simulink subsystem "DCDCConverter"  (R2024b)
settings: Solver=VariableStepAuto  StartTime=0.0  StopTime=10.0  RelTol=1e-3
undefined symbols (not defined in the file): PlntDCDCMass, PlntDCDCVoltInit, PlntEMCp
libraries: autolibutils x1, autolibdcdc x1, autolibsharedcommon x1
settings Model: ModifiedByFormat=The MathWorks, Inc.  Creator=The MathWorks, Inc.  LastModifiedBy=The MathWorks, Inc.
settings OptimizationCC: ReuseModelBlockBuffer=off
settings RTWCC: GPUComputeCapability=3.5

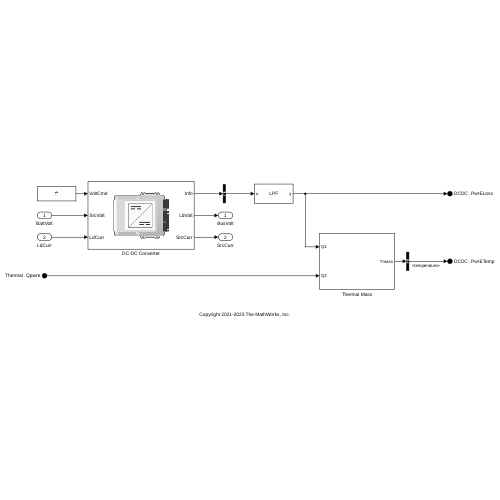
[thumbnail: Simulink's stored preview of the top-level diagram]
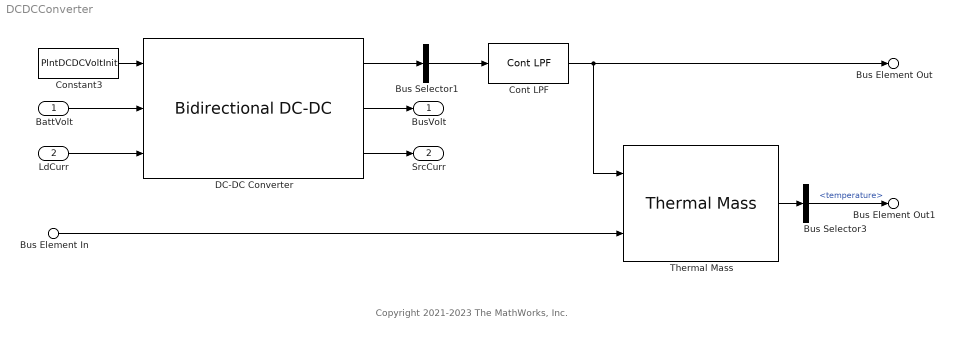
== system DCDCConverter ==
  note: Copyright 2021-2023 The MathWorks, Inc.
  BattVolt : Inport
  LdCurr : Inport  Port=2
  Bus Element In : Inport  Port=3  PortName=Thermal  Element=Qpwre
  Bus Selector1 : BusSelector  OutputSignals=PwrLoss  OutputAsBus=on
  Bus Selector3 : BusSelector  OutputSignals=temperature
  Constant3 : Constant  Value=PlntDCDCVoltInit  SampleTime=-1
  Cont LPF : autolibutils/Cont LPF  wc=1  AbsoluteTolerance=auto  aMode=6
  DC-DC Converter : autolibdcdc/Bidirectional DC-DC  Tc=PlntDCDCTimeCnst  Vinit=PlntDCDCVoltInit  Plimit=PlntDCDCPwrLmt  param_loss=Single efficiency measurement  eff=PlntDCDCEff  v_loss_bp=PlntDCDCLossV  i_loss_bp=PlntDCDCLossI  losses_table=PlntDCDCLossTbl  v_eff_bp=[200 400 600 800 1000]  i_eff_bp=[25 50 75 100]  efficiency_table=[96.2 98.1 98.7 99;98.1 99 99.4 99.5;98.7 99.4 99.6 99.7;99 99.5 99.7 99.8;99.2 99.6 99.7 99.8]  x_v_bp=[-1000 -800 -600 -400 -200 200 400 600 800 1000]  x_i_bp=[-100 -75 -50 -25 25 50 75 100]  x_losses_mat=[200.400801603196 225.67703109328 200.803212851408 201.612903225806 199.999999999997 200 225 200;160.320641282556 180.541624874624 201.005025125625 202.020202020203 200 200 180 160;180.541624874624 180.722891566267 181.086519114686 197.568389057748 194.999999999999 179.999999999997 180 180;201.005025125625 181.086519114686 202.020202020203 193.67991845056 190 200 179.999999999997 200;202.020202020203 197.568389057748 193.67991845056 197.505197505197 190 190 194.999999999999 200;200 194.999999999999 190 190 197.505197505197 193.67991845056 197.568389057748 202.020202020203;200 179.999999999997 200 190 193.67991845056 202.020202020203 181.086519114686 201.005025125625;180 180 179.999999999997 194.999999999999 197.568389057748 181.086519114686 180.722891566267 180.541624874624;160 180 200 200 202.020202020203 201.005025125625 180.541624874624 160.320641282556;200 225 200 199.999999999997 201.612903225806 200.803212851408 225.67703109328 200.400801603196]  RefBlkName='autolibdcdc/Bidirectional DC-DC'  CalLossMapData={'BaseCageProjectFileName','';'BaseMbcProjectFileName','';'TaskName','Calibrate Inverter Loss Map';'ChildTasks',{{'DataName','';'TaskName','Import Loss Data'},{'TaskName','Generate Response Models'},{'TaskName','Generate Calibration'},{'TaskName','Update Block Parameters'}}}
  Thermal Mass : autolibsharedcommon/Thermal Mass  MassOrVol=Mass  Mass=PlntDCDCMass  Volume=10  Rho=997  HeatCp=PlntEMCp*ones(1,2)  HeatBrkPts=PlntBattCpBpt  Tinit=EnvAirTemp  Tenv=EnvAirTemp  ConvHTC=1  EnvArea=0.1
  BusVolt : Outport  VectorParamsAs1DForOutWhenUnconnected=off
  SrcCurr : Outport  Port=2  VectorParamsAs1DForOutWhenUnconnected=off
  Bus Element Out : Outport  Port=3  PortName=DCDC  Element=PwrELoss
  Bus Element Out1 : Outport  Port=3  PortName=DCDC  Element=PwrETemp
  wires:
  Constant3/1 -> DC-DC Converter/1
  DC-DC Converter/3 -> SrcCurr/1
  DC-DC Converter/1 -> Bus Selector1/1
  BattVolt/1 -> DC-DC Converter/2
  DC-DC Converter/2 -> BusVolt/1
  LdCurr/1 -> DC-DC Converter/3
  Bus Selector1/1 -> Cont LPF/1
  Cont LPF/1 -> Bus Element Out/1, Thermal Mass/1
  Bus Element In/1 -> Thermal Mass/2
  Thermal Mass/1 -> Bus Selector3/1
  Bus Selector3/1 -> Bus Element Out1/1  "<temperature>"
